simulink model "deneme"  (R2022a)
settings: Solver=VariableStepAuto  StartTime=0.0  StopTime=10.0  RelTol=1e-3
model workspace (MAT data in the model file):
  L = 1.756
  g = 9.80665
settings Model: Creator=gkonu  LastModifiedBy=asimg

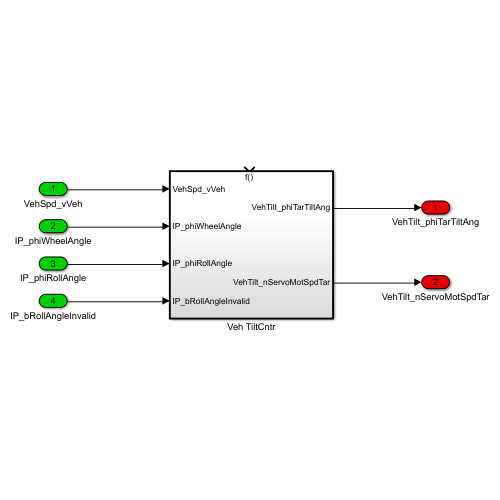
[thumbnail: Simulink's stored preview of the top-level diagram]
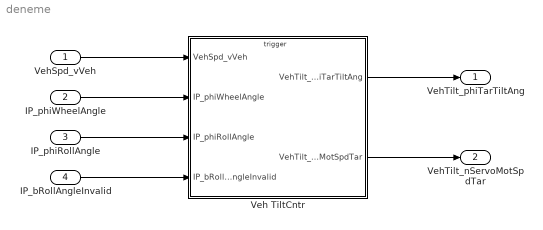
== system deneme ==
  VehSpd_vVeh : Inport
  IP_phiWheelAngle : Inport  Port=2
  IP_phiRollAngle : Inport  Port=3
  IP_bRollAngleInvalid : Inport  Port=4
  Veh TiltCntr : Subsystem
  VehTilt_phiTarTiltAng : Outport
  VehTilt_nServoMotSpdTar : Outport  Port=2
  wires:
  Veh TiltCntr/2(VehTilt_nServoMotSpdTar) -> VehTilt_nServoMotSpdTar/1
  VehSpd_vVeh/1 -> Veh TiltCntr/1(VehSpd_vVeh)
  IP_phiRollAngle/1 -> Veh TiltCntr/3(IP_phiRollAngle)
  Veh TiltCntr/1(VehTilt_phiTarTiltAng) -> VehTilt_phiTarTiltAng/1
  IP_bRollAngleInvalid/1 -> Veh TiltCntr/4(IP_bRollAngleInvalid)
  IP_phiWheelAngle/1 -> Veh TiltCntr/2(IP_phiWheelAngle)

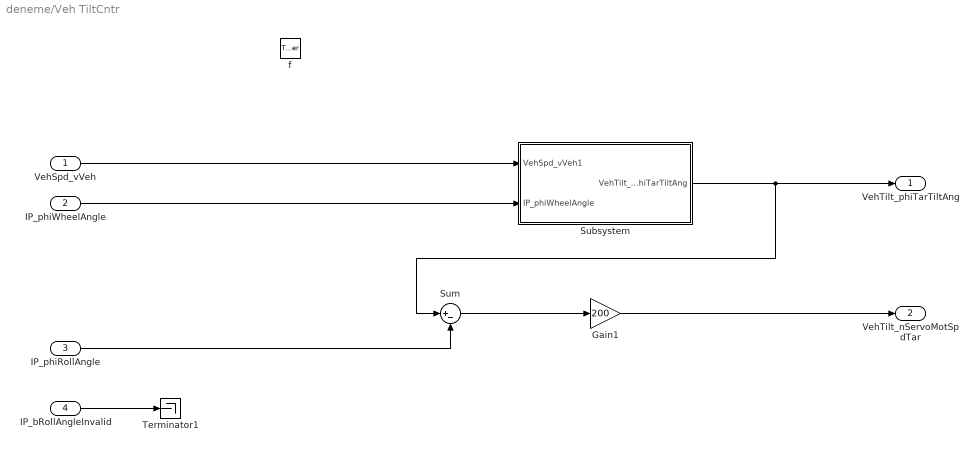
== system deneme/Veh TiltCntr ==
  VehSpd_vVeh : Inport
  IP_phiWheelAngle : Inport  Port=2
  IP_phiRollAngle : Inport  Port=3
  IP_bRollAngleInvalid : Inport  Port=4
  f : TriggerPort  TriggerType=function-call  VariantControl=(inherit)
  Gain1 : Gain  Gain=200
  Subsystem : Subsystem
  Sum : Sum  Inputs=|+-
  Terminator1 : Terminator
  VehTilt_phiTarTiltAng : Outport
  VehTilt_nServoMotSpdTar : Outport  Port=2
  wires:
  VehSpd_vVeh/1 -> Subsystem/1(VehSpd_vVeh1)
  IP_phiRollAngle/1 -> Sum/2
  IP_bRollAngleInvalid/1 -> Terminator1/1
  Sum/1 -> Gain1/1
  Gain1/1 -> VehTilt_nServoMotSpdTar/1
  Subsystem/1(VehTilt_phiTarTiltAng) -> VehTilt_phiTarTiltAng/1, Sum/1
  IP_phiWheelAngle/1 -> Subsystem/2(IP_phiWheelAngle)

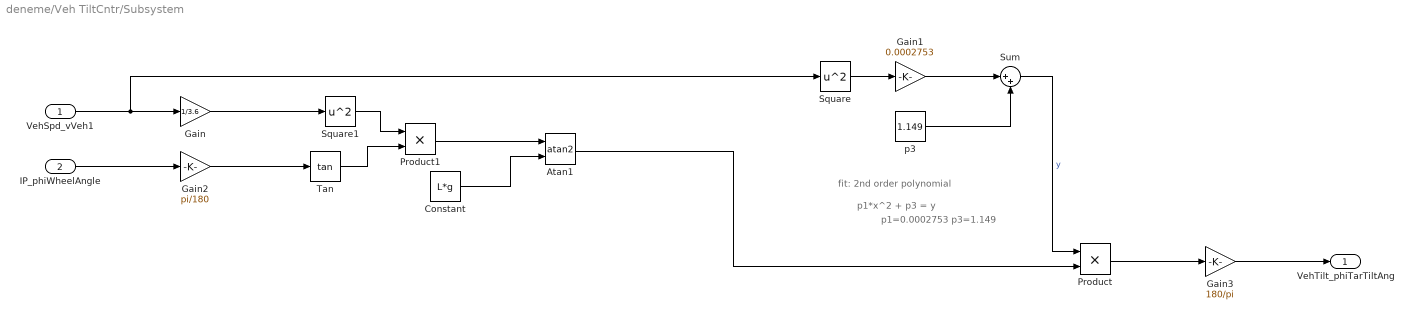
== system deneme/Veh TiltCntr/Subsystem ==
  note: p1*x^2 + p3 = y
  note: p1=0.0002753
      | p3=1.149
  note: fit: 2nd order polynomial
  VehSpd_vVeh1 : Inport
  IP_phiWheelAngle : Inport  Port=2
  Atan1 : Trigonometry  Operator=atan2
  Constant : Constant  Value=L*g
  Gain : Gain  Gain=1/3.6
  Gain1 : Gain  Gain=0.0002753
  Gain2 : Gain  Gain=pi/180
  Gain3 : Gain  Gain=180/pi
  Product : Product
  Product1 : Product
  Square : Math  Operator=square
  Square1 : Math  Operator=square
  Sum : Sum  Inputs=|++
  Tan : Trigonometry  Operator=tan
  p3 : Constant  Value=1.149
  VehTilt_phiTarTiltAng : Outport
  wires:
  VehSpd_vVeh1/1 -> Square/1, Gain/1
  Square/1 -> Gain1/1
  p3/1 -> Sum/2
  Gain1/1 -> Sum/1
  Sum/1 -> Product/1  "y"
  Atan1/1 -> Product/2
  Product/1 -> Gain3/1
  Product1/1 -> Atan1/1
  Square1/1 -> Product1/1
  Constant/1 -> Atan1/2
  Tan/1 -> Product1/2
  IP_phiWheelAngle/1 -> Gain2/1
  Gain/1 -> Square1/1
  Gain2/1 -> Tan/1
  Gain3/1 -> VehTilt_phiTarTiltAng/1
